simulink subsystem "distance_magnitude_3D"  (R2023a)
settings: Solver=VariableStepAuto  StartTime=0.0  StopTime=10.0  RelTol=1e-3
undefined symbols (not defined in the file): magnitude
settings Model: Creator=bjmyn  LastModifiedBy=bjmyn

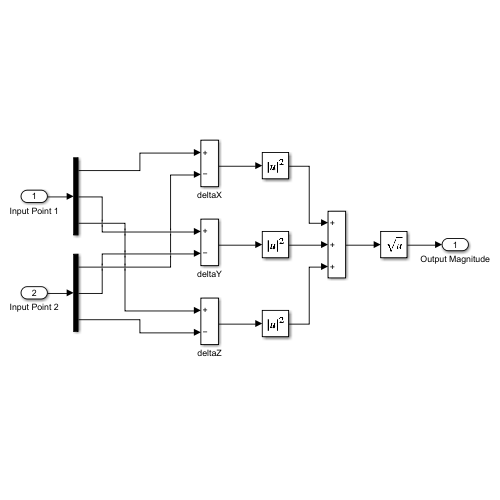
[thumbnail: Simulink's stored preview of the top-level diagram]
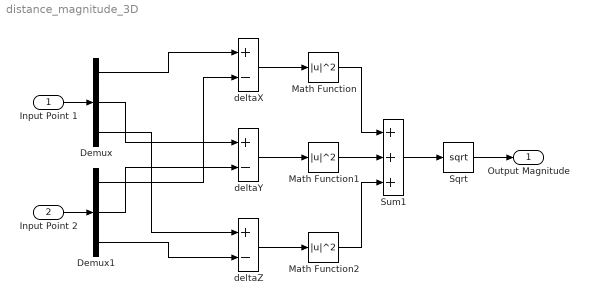
== system distance_magnitude_3D ==
  Input Point 1 : Inport
  Input Point 2 : Inport  Port=2
  Demux : Demux  Outputs=3
  Demux1 : Demux  Outputs=3
  Math Function : Math  Operator=magnitude^2
  Math Function1 : Math  Operator=magnitude^2
  Math Function2 : Math  Operator=magnitude^2
  Sqrt : Sqrt
  Sum1 : Sum  Inputs=+++
  deltaX : Sum  Inputs=+-
  deltaY : Sum  Inputs=+-
  deltaZ : Sum  Inputs=+-
  Output Magnitude : Outport
  wires:
  Input Point 1/1 -> Demux/1
  Input Point 2/1 -> Demux1/1
  deltaX/1 -> Math Function/1
  Sum1/1 -> Sqrt/1
  Math Function/1 -> Sum1/1
  Demux/1 -> deltaX/1
  Demux1/1 -> deltaX/2
  deltaY/1 -> Math Function1/1
  deltaZ/1 -> Math Function2/1
  Demux1/3 -> deltaZ/2
  Demux/3 -> deltaZ/1
  Demux1/2 -> deltaY/2
  Demux/2 -> deltaY/1
  Math Function1/1 -> Sum1/2
  Math Function2/1 -> Sum1/3
  Sqrt/1 -> Output Magnitude/1
